simulink library "ODEsim"  (R2024b)
settings: Solver=VariableStepAuto  StartTime=0.0  StopTime=10.0  RelTol=1e-3
undefined symbols (not defined in the file or in its folder): Cline_2, Cline_r_2, Cout_9, Fb_18, Fb_d_18, fs_9, K_d_18, Ki_18, Ki_4, Kp_18, Kp_4, Len_2, R_4, r_C, r_C_1, Rline_2, Rload, Td_18, Td_4
libraries: fl_lib x97, ee_lib x24, nesl_utility x20, simulink_extras x2, spsSawtoothGeneratorLib x2, simulink x2
(part 2 of 2)

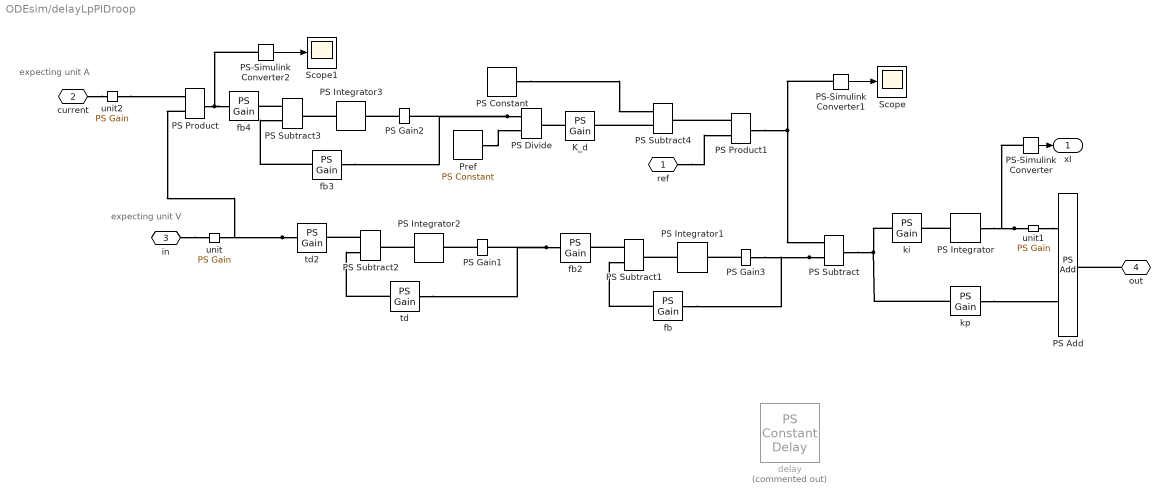
== system ODEsim/delayLpPIDroop ==
  note: expecting unit A
  note: expecting unit V
  K_d : fl_lib/Physical Signals/Functions/PS Gain  gain=K_d_18
  PS Add : fl_lib/Physical Signals/Functions/PS Add
  PS Constant : fl_lib/Physical Signals/Sources/PS Constant  constant=1
  PS Divide : fl_lib/Physical Signals/Functions/PS Divide
  PS Gain1 : fl_lib/Physical Signals/Functions/PS Gain  gain=1 1/s
  PS Gain2 : fl_lib/Physical Signals/Functions/PS Gain  gain=1 1/s
  PS Gain3 : fl_lib/Physical Signals/Functions/PS Gain  gain=1 1/s
  PS Integrator : fl_lib/Physical Signals/Linear Operators/PS Integrator  reset_method=foundation.enum.IntegratorResetSpec.None  initial_condition_spec=foundation.enum.IntegratorICSpec.Internal  saturation_spec=foundation.enum.IntegratorSaturationSpec.Both  saturation_source_spec=foundation.enum.IntegratorSaturationSourceSpec.Internal  x0=0 s  xu=90 s  xl=-0 s
  PS Integrator1 : fl_lib/Physical Signals/Linear Operators/PS Integrator  reset_method=foundation.enum.IntegratorResetSpec.None  initial_condition_spec=foundation.enum.IntegratorICSpec.Internal  saturation_spec=foundation.enum.IntegratorSaturationSpec.None  saturation_source_spec=foundation.enum.IntegratorSaturationSourceSpec.Internal  x0=0 s  xu=inf s  xl=-inf s
  PS Integrator2 : fl_lib/Physical Signals/Linear Operators/PS Integrator  reset_method=foundation.enum.IntegratorResetSpec.None  initial_condition_spec=foundation.enum.IntegratorICSpec.Internal  saturation_spec=foundation.enum.IntegratorSaturationSpec.None  saturation_source_spec=foundation.enum.IntegratorSaturationSourceSpec.Internal  x0=0 s  xu=inf s  xl=-inf s
  PS Integrator3 : fl_lib/Physical Signals/Linear Operators/PS Integrator  reset_method=foundation.enum.IntegratorResetSpec.None  initial_condition_spec=foundation.enum.IntegratorICSpec.Internal  saturation_spec=foundation.enum.IntegratorSaturationSpec.None  saturation_source_spec=foundation.enum.IntegratorSaturationSourceSpec.Internal  x0=0 s  xu=inf s  xl=-inf s
  PS Product : fl_lib/Physical Signals/Functions/PS Product
  PS Product1 : fl_lib/Physical Signals/Functions/PS Product
  PS Subtract{,1..4} (5 alike) : fl_lib/Physical Signals/Functions/PS Subtract
  PS-Simulink Converter : nesl_utility/PS-Simulink Converter  PhysicalDomain=network_engine_domain  SubClassName=ps_output  LeftPortType=input  RightPortType=output  PseudoPeriodic=off  Frequencies=[]  VectorFormat=inherit  Unit=inherit  AffineConversion=off
  PS-Simulink Converter1 : nesl_utility/PS-Simulink Converter  PhysicalDomain=network_engine_domain  SubClassName=ps_output  LeftPortType=input  RightPortType=output  PseudoPeriodic=off  Frequencies=[]  VectorFormat=inherit  Unit=inherit  AffineConversion=off
  PS-Simulink Converter2 : nesl_utility/PS-Simulink Converter  PhysicalDomain=network_engine_domain  SubClassName=ps_output  LeftPortType=input  RightPortType=output  PseudoPeriodic=off  Frequencies=[]  VectorFormat=inherit  Unit=inherit  AffineConversion=off
  Pref : fl_lib/Physical Signals/Sources/PS Constant  constant=P_d_18
  Scope : Scope
  Scope1 : Scope
  delay : fl_lib/Physical Signals/Delays/PS Constant Delay  Commented=on  InputHistory=0.0  DelayTime=Td_4 s
      settings: InternalSimscapePortConfiguration="{\"Bottom\":[],\"Left\":[{\"id\":\"U\",\"label\":\"U\",\"type\":\"input\"}],\"Right\":[{\"id\":\"Y\",\"label\":\"Y\",\"type\":\"output\"}],\"Top\":[]}"
  fb : fl_lib/Physical Signals/Functions/PS Gain  gain=2*pi*Fb_18
  fb2 : fl_lib/Physical Signals/Functions/PS Gain  gain=2*pi*Fb_18
  fb3 : fl_lib/Physical Signals/Functions/PS Gain  gain=Fb_d_18* 2 * pi
  fb4 : fl_lib/Physical Signals/Functions/PS Gain  gain=Fb_d_18* 2 * pi
  ki : fl_lib/Physical Signals/Functions/PS Gain  gain=Ki_18
  kp : fl_lib/Physical Signals/Functions/PS Gain  gain=Kp_18
  td : fl_lib/Physical Signals/Functions/PS Gain  gain=1/Td_18
  td2 : fl_lib/Physical Signals/Functions/PS Gain  gain=1/Td_18
  unit : fl_lib/Physical Signals/Functions/PS Gain  gain=1 1/V
  unit1 : fl_lib/Physical Signals/Functions/PS Gain  gain=1 1/s
  unit2 : fl_lib/Physical Signals/Functions/PS Gain  gain=1 1/A
  ref : PMIOPort  Side=Left
  current : PMIOPort  Port=2  Side=Left
  in : PMIOPort  Port=3  Side=Left
  out : PMIOPort  Port=4  Side=Right
  xI : Outport
  wires:
  PS-Simulink Converter/1 -> xI/1
  PS-Simulink Converter1/1 -> Scope/1
  PS-Simulink Converter2/1 -> Scope1/1
  connections:
  PS Subtract4/LConn2 -- K_d/RConn1
  PS Product1/RConn1 -- PS Subtract/LConn1 -- PS-Simulink Converter1/LConn1
  ref/RConn1 -- PS Product1/LConn2
  PS Product1/LConn1 -- PS Subtract4/RConn1
  Pref/RConn1 -- PS Divide/LConn2
  PS Constant/RConn1 -- PS Subtract4/LConn1
  K_d/LConn1 -- PS Divide/RConn1
  unit2/RConn1 -- PS Product/LConn1
  current/RConn1 -- unit2/LConn1
  fb3/RConn1 -- PS Subtract3/LConn2
  PS Subtract3/LConn1 -- fb4/RConn1
  PS Integrator3/LConn1 -- PS Subtract3/RConn1
  PS Gain2/LConn1 -- PS Integrator3/RConn1
  PS Product/RConn1 -- PS-Simulink Converter2/LConn1 -- fb4/LConn1
  PS Divide/LConn1 -- PS Gain2/RConn1 -- fb3/LConn1
  td/RConn1 -- PS Subtract2/LConn2
  PS Integrator2/LConn1 -- PS Subtract2/RConn1
  PS Subtract2/LConn1 -- td2/RConn1
  PS Gain1/LConn1 -- PS Integrator2/RConn1
  td2/LConn1 -- unit/RConn1 -- PS Product/LConn2
  fb2/LConn1 -- PS Gain1/RConn1 -- td/LConn1
  unit1/RConn1 -- PS Add/LConn1
  PS Subtract/RConn1 -- kp/LConn1 -- ki/LConn1
  PS Integrator/LConn1 -- ki/RConn1
  in/RConn1 -- unit/LConn1
  unit1/LConn1 -- PS Integrator/RConn1 -- PS-Simulink Converter/LConn1
  kp/RConn1 -- PS Add/LConn2
  out/RConn1 -- PS Add/RConn1
  PS Subtract/LConn2 -- PS Gain3/RConn1 -- fb/LConn1
  fb/RConn1 -- PS Subtract1/LConn2
  PS Integrator1/LConn1 -- PS Subtract1/RConn1
  PS Subtract1/LConn1 -- fb2/RConn1
  PS Gain3/LConn1 -- PS Integrator1/RConn1

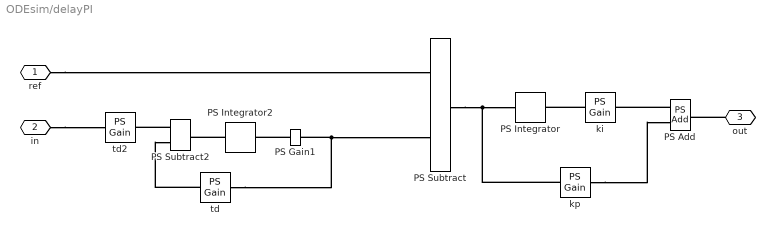
== system ODEsim/delayPI ==
  PS Add : fl_lib/Physical Signals/Functions/PS Add
  PS Gain1 : fl_lib/Physical Signals/Functions/PS Gain  gain=1 1/s
  PS Integrator : fl_lib/Physical Signals/Linear Operators/PS Integrator  reset_method=foundation.enum.IntegratorResetSpec.None  initial_condition_spec=foundation.enum.IntegratorICSpec.Internal  saturation_spec=foundation.enum.IntegratorSaturationSpec.None  saturation_source_spec=foundation.enum.IntegratorSaturationSourceSpec.Internal  x0=0 s  xu=inf s  xl=-inf s
  PS Integrator2 : fl_lib/Physical Signals/Linear Operators/PS Integrator  reset_method=foundation.enum.IntegratorResetSpec.None  initial_condition_spec=foundation.enum.IntegratorICSpec.Internal  saturation_spec=foundation.enum.IntegratorSaturationSpec.None  saturation_source_spec=foundation.enum.IntegratorSaturationSourceSpec.Internal  x0=0 s  xu=inf s  xl=-inf s
  PS Subtract : fl_lib/Physical Signals/Functions/PS Subtract
  PS Subtract2 : fl_lib/Physical Signals/Functions/PS Subtract
  ki : fl_lib/Physical Signals/Functions/PS Gain  gain=Ki_4 1/s
  kp : fl_lib/Physical Signals/Functions/PS Gain  gain=Kp_4
  td : fl_lib/Physical Signals/Functions/PS Gain  gain=1/Td_18
  td2 : fl_lib/Physical Signals/Functions/PS Gain  gain=1/Td_18
  ref : PMIOPort  Side=Left
  in : PMIOPort  Port=2  Side=Left
  out : PMIOPort  Port=3  Side=Right
  connections:
  out/RConn1 -- PS Add/RConn1
  kp/RConn1 -- PS Add/LConn2
  ki/LConn1 -- PS Integrator/RConn1
  PS Add/LConn1 -- ki/RConn1
  in/RConn1 -- td2/LConn1
  td/LConn1 -- PS Subtract/LConn2 -- PS Gain1/RConn1
  ref/RConn1 -- PS Subtract/LConn1
  PS Subtract/RConn1 -- kp/LConn1 -- PS Integrator/LConn1
  td/RConn1 -- PS Subtract2/LConn2
  PS Subtract2/LConn1 -- td2/RConn1
  PS Integrator2/LConn1 -- PS Subtract2/RConn1
  PS Gain1/LConn1 -- PS Integrator2/RConn1

== system ODEsim/loadRL ==
  Lload : ee_lib/Passive/Inductor  l=Lload H  enable_L_tol=ee.enum.toleranceApplication.none  L_tol=20  tol_distribution=ee.enum.toleranceDistribution.uniform  nSigma=4  r=0 Ohm  g=0 1/Ohm  enable_operating_limits=ee.enum.enable.no  operating_limit_action=ee.enum.passive.reportOpLim.warn  max_working_current=1 A  power_rating=1 W  fault_action=simscape.enum.assert.action.none  t_fault=1 s  i_L_specify=off  i_L_priority=High  i_L=0 A  i_L_nominal_specify=off  i_L_nominal_value=1  i_L_nominal_unit=A
  M : Subsystem
      settings: CopyFcn=set_param(gcb,'LinkStatus','none')  PortSchema="{\"entries\":[{\"content\":{\"sides\":[{\"content\":{\"connectorIds\":[\"LConn1\"]},\"type\":\"ConnectorPlacement.EquallySpacedRectSide\",\"uuid\":\"40852030-531f-4f43-a55b-e3170444f81a\"},{\"content\":{\"connectorIds\":[\"RConn1\"],\"side\":\"RIGHT\"},\"type\":\"ConnectorPlacement.EquallySpacedRectSide\",\"uuid\":\"1f30083b-b568-47ae-a4c9-b443d22c2592\"},{\"content\":{\"connectorIds\":[\"LConn2\"],\"side\":\"TOP\"},\"type\":\"ConnectorPlacement.EquallySpacedRectSide\",\"uuid\":\"3c071041-7a52-4d22-9e74-6a603f214a57\"}]},\"type\":\"ConnectorPlacement.EquallySpacedConnector\",\"uuid\":\"06d852a0-3ad3-4e59-bc5b-9ea8903862cb\"}],\"packageUris\":[\"http://schema.mathworks.com/mf0/Connector/R2020b\"],\"version\":\"1.0\"}"
  Rload : fl_lib/Electrical/Electrical Elements/Resistor  R=Rload Ohm  i_specify=off  i_priority=None  i=0 A  i_nominal_specify=off  i_nominal_value=1  i_nominal_unit=A  v_specify=off  v_priority=None  v=0 V  v_nominal_specify=off  v_nominal_value=1  v_nominal_unit=V
  In : PMIOPort  Side=Left
  Gnd : PMIOPort  Port=2  Side=Left
  i_L : PMIOPort  Port=3  Side=Left
  connections:
  Gnd/RConn1 -- M/RConn1
  Rload/LConn1 -- In/RConn1
  M/LConn1 -- Lload/RConn1
  Rload/RConn1 -- Lload/LConn1
  i_L/RConn1 -- M/LConn2

== system ODEsim/loadVarRL ==
  Lload : ee_lib/Passive/Inductor  l=Lload_3 H  enable_L_tol=ee.enum.toleranceApplication.none  L_tol=20  tol_distribution=ee.enum.toleranceDistribution.uniform  nSigma=4  r=0 Ohm  g=0 1/Ohm  enable_operating_limits=ee.enum.enable.no  operating_limit_action=ee.enum.passive.reportOpLim.warn  max_working_current=1 A  power_rating=1 W  fault_action=simscape.enum.assert.action.none  t_fault=1 s  i_L_specify=off  i_L_priority=High  i_L=0 A  i_L_nominal_specify=off  i_L_nominal_value=1  i_L_nominal_unit=A
  M : Subsystem
      settings: CopyFcn=set_param(gcb,'LinkStatus','none')  PortSchema="{\"entries\":[{\"content\":{\"sides\":[{\"content\":{\"connectorIds\":[\"LConn1\"]},\"type\":\"ConnectorPlacement.EquallySpacedRectSide\",\"uuid\":\"40852030-531f-4f43-a55b-e3170444f81a\"},{\"content\":{\"connectorIds\":[\"RConn1\"],\"side\":\"RIGHT\"},\"type\":\"ConnectorPlacement.EquallySpacedRectSide\",\"uuid\":\"1f30083b-b568-47ae-a4c9-b443d22c2592\"},{\"content\":{\"connectorIds\":[\"LConn2\"],\"side\":\"TOP\"},\"type\":\"ConnectorPlacement.EquallySpacedRectSide\",\"uuid\":\"3c071041-7a52-4d22-9e74-6a603f214a57\"}]},\"type\":\"ConnectorPlacement.EquallySpacedConnector\",\"uuid\":\"06d852a0-3ad3-4e59-bc5b-9ea8903862cb\"}],\"packageUris\":[\"http://schema.mathworks.com/mf0/Connector/R2020b\"],\"version\":\"1.0\"}"
  Variable Resistor : fl_lib/Electrical/Electrical Elements/Variable Resistor  Rmin=0 Ohm  thermalEnable=false  thermal_mass=1 J/K  i_specify=off  i_priority=None  i=0 A  i_nominal_specify=off  i_nominal_value=1  i_nominal_unit=A  v_specify=off  v_priority=None  v=0 V  v_nominal_specify=off  v_nominal_value=1  v_nominal_unit=V  T_specify=off  T_priority=None  T=300 K  T_nominal_specify=off  T_nominal_value=1  T_nominal_unit=K
  In : PMIOPort  Side=Left
  Gnd : PMIOPort  Port=2  Side=Left
  i_L : PMIOPort  Port=3  Side=Left
  R : PMIOPort  Port=4  Side=Right
  connections:
  Lload/LConn1 -- Variable Resistor/RConn1
  Lload/RConn1 -- M/LConn1
  R/RConn1 -- Variable Resistor/LConn1
  In/RConn1 -- Variable Resistor/LConn2
  M/RConn1 -- Gnd/RConn1
  i_L/RConn1 -- M/LConn2

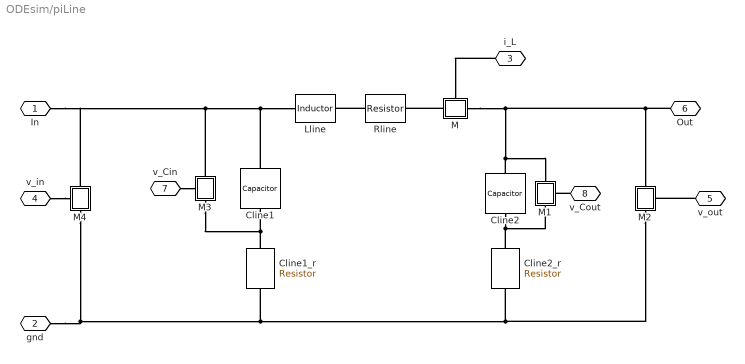
== system ODEsim/piLine ==
  Cline1 : fl_lib/Electrical/Electrical Elements/Capacitor  c=Cline_2 / 2 *Len_2 F  r=0 Ohm  g=0 1/Ohm  i_specify=off  i_priority=None  i=0 A  i_nominal_specify=off  i_nominal_value=1  i_nominal_unit=A  v_specify=off  v_priority=None  v=0 V  v_nominal_specify=off  v_nominal_value=1  v_nominal_unit=V  vc_specify=off  vc_priority=High  vc=0 V  vc_nominal_specify=off  vc_nominal_value=1  vc_nominal_unit=V
  Cline1_r : fl_lib/Electrical/Electrical Elements/Resistor  R=Cline_r_2 Ohm  i_specify=off  i_priority=None  i=0 A  i_nominal_specify=off  i_nominal_value=1  i_nominal_unit=A  v_specify=off  v_priority=None  v=0 V  v_nominal_specify=off  v_nominal_value=1  v_nominal_unit=V
  Cline2 : fl_lib/Electrical/Electrical Elements/Capacitor  c=Cline_2 / 2 *Len_2 F  r=0 Ohm  g=0 1/Ohm  i_specify=off  i_priority=None  i=0 A  i_nominal_specify=off  i_nominal_value=1  i_nominal_unit=A  v_specify=off  v_priority=None  v=0 V  v_nominal_specify=off  v_nominal_value=1  v_nominal_unit=V  vc_specify=off  vc_priority=High  vc=0 V  vc_nominal_specify=off  vc_nominal_value=1  vc_nominal_unit=V
  Cline2_r : fl_lib/Electrical/Electrical Elements/Resistor  R=Cline_r_2 Ohm  i_specify=off  i_priority=None  i=0 A  i_nominal_specify=off  i_nominal_value=1  i_nominal_unit=A  v_specify=off  v_priority=None  v=0 V  v_nominal_specify=off  v_nominal_value=1  v_nominal_unit=V
  Lline : fl_lib/Electrical/Electrical Elements/Inductor  l=Lline_2 H  r=0 Ohm  g=0 1/Ohm  i_specify=off  i_priority=None  i=0 A  i_nominal_specify=off  i_nominal_value=1  i_nominal_unit=A  v_specify=off  v_priority=None  v=0 V  v_nominal_specify=off  v_nominal_value=1  v_nominal_unit=V  i_L_specify=off  i_L_priority=High  i_L=0 A  i_L_nominal_specify=off  i_L_nominal_value=1  i_L_nominal_unit=A
  M : Subsystem
      settings: CopyFcn=set_param(gcb,'LinkStatus','none')  PortSchema="{\"entries\":[{\"content\":{\"sides\":[{\"content\":{\"connectorIds\":[\"LConn1\"]},\"type\":\"ConnectorPlacement.EquallySpacedRectSide\",\"uuid\":\"40852030-531f-4f43-a55b-e3170444f81a\"},{\"content\":{\"connectorIds\":[\"RConn1\"],\"side\":\"RIGHT\"},\"type\":\"ConnectorPlacement.EquallySpacedRectSide\",\"uuid\":\"1f30083b-b568-47ae-a4c9-b443d22c2592\"},{\"content\":{\"connectorIds\":[\"LConn2\"],\"side\":\"TOP\"},\"type\":\"ConnectorPlacement.EquallySpacedRectSide\",\"uuid\":\"3c071041-7a52-4d22-9e74-6a603f214a57\"}]},\"type\":\"ConnectorPlacement.EquallySpacedConnector\",\"uuid\":\"06d852a0-3ad3-4e59-bc5b-9ea8903862cb\"}],\"packageUris\":[\"http://schema.mathworks.com/mf0/Connector/R2020b\"],\"version\":\"1.0\"}"
  M1 : Subsystem
      settings: CopyFcn=set_param(gcb,'LinkStatus','none')  PortSchema="{\"entries\":[{\"content\":{\"sides\":[{\"content\":{\"connectorIds\":[\"LConn1\"]},\"type\":\"ConnectorPlacement.EquallySpacedRectSide\",\"uuid\":\"06c3c841-7f27-414f-b368-a176494b6f9d\"},{\"content\":{\"connectorIds\":[\"RConn1\"],\"side\":\"RIGHT\"},\"type\":\"ConnectorPlacement.EquallySpacedRectSide\",\"uuid\":\"1b123208-a0a4-432d-8d9c-871fed45b507\"},{\"content\":{\"connectorIds\":[\"LConn2\"],\"side\":\"TOP\"},\"type\":\"ConnectorPlacement.EquallySpacedRectSide\",\"uuid\":\"cfe0dd68-fe1a-447a-9562-3abbfb037eea\"}]},\"type\":\"ConnectorPlacement.EquallySpacedConnector\",\"uuid\":\"2a5dcc2a-148a-4bfc-a97a-46b06b110d1b\"}],\"packageUris\":[\"http://schema.mathworks.com/mf0/Connector/R2020b\"],\"version\":\"1.0\"}"
  M2 : Subsystem
      settings: CopyFcn=set_param(gcb,'LinkStatus','none')  PortSchema="{\"entries\":[{\"content\":{\"sides\":[{\"content\":{\"connectorIds\":[\"LConn1\"]},\"type\":\"ConnectorPlacement.EquallySpacedRectSide\",\"uuid\":\"06c3c841-7f27-414f-b368-a176494b6f9d\"},{\"content\":{\"connectorIds\":[\"RConn1\"],\"side\":\"RIGHT\"},\"type\":\"ConnectorPlacement.EquallySpacedRectSide\",\"uuid\":\"1b123208-a0a4-432d-8d9c-871fed45b507\"},{\"content\":{\"connectorIds\":[\"LConn2\"],\"side\":\"TOP\"},\"type\":\"ConnectorPlacement.EquallySpacedRectSide\",\"uuid\":\"cfe0dd68-fe1a-447a-9562-3abbfb037eea\"}]},\"type\":\"ConnectorPlacement.EquallySpacedConnector\",\"uuid\":\"2a5dcc2a-148a-4bfc-a97a-46b06b110d1b\"}],\"packageUris\":[\"http://schema.mathworks.com/mf0/Connector/R2020b\"],\"version\":\"1.0\"}"
  M3 : Subsystem
      settings: CopyFcn=set_param(gcb,'LinkStatus','none')  PortSchema="{\"entries\":[{\"content\":{\"sides\":[{\"content\":{\"connectorIds\":[\"LConn1\"]},\"type\":\"ConnectorPlacement.EquallySpacedRectSide\",\"uuid\":\"06c3c841-7f27-414f-b368-a176494b6f9d\"},{\"content\":{\"connectorIds\":[\"RConn1\"],\"side\":\"RIGHT\"},\"type\":\"ConnectorPlacement.EquallySpacedRectSide\",\"uuid\":\"1b123208-a0a4-432d-8d9c-871fed45b507\"},{\"content\":{\"connectorIds\":[\"LConn2\"],\"side\":\"TOP\"},\"type\":\"ConnectorPlacement.EquallySpacedRectSide\",\"uuid\":\"cfe0dd68-fe1a-447a-9562-3abbfb037eea\"}]},\"type\":\"ConnectorPlacement.EquallySpacedConnector\",\"uuid\":\"2a5dcc2a-148a-4bfc-a97a-46b06b110d1b\"}],\"packageUris\":[\"http://schema.mathworks.com/mf0/Connector/R2020b\"],\"version\":\"1.0\"}"
  M4 : Subsystem
      settings: CopyFcn=set_param(gcb,'LinkStatus','none')  PortSchema="{\"entries\":[{\"content\":{\"sides\":[{\"content\":{\"connectorIds\":[\"LConn1\"]},\"type\":\"ConnectorPlacement.EquallySpacedRectSide\",\"uuid\":\"06c3c841-7f27-414f-b368-a176494b6f9d\"},{\"content\":{\"connectorIds\":[\"RConn1\"],\"side\":\"RIGHT\"},\"type\":\"ConnectorPlacement.EquallySpacedRectSide\",\"uuid\":\"1b123208-a0a4-432d-8d9c-871fed45b507\"},{\"content\":{\"connectorIds\":[\"LConn2\"],\"side\":\"TOP\"},\"type\":\"ConnectorPlacement.EquallySpacedRectSide\",\"uuid\":\"cfe0dd68-fe1a-447a-9562-3abbfb037eea\"}]},\"type\":\"ConnectorPlacement.EquallySpacedConnector\",\"uuid\":\"2a5dcc2a-148a-4bfc-a97a-46b06b110d1b\"}],\"packageUris\":[\"http://schema.mathworks.com/mf0/Connector/R2020b\"],\"version\":\"1.0\"}"
  Rline : fl_lib/Electrical/Electrical Elements/Resistor  R=Rline_2 Ohm  i_specify=off  i_priority=None  i=0 A  i_nominal_specify=off  i_nominal_value=1  i_nominal_unit=A  v_specify=off  v_priority=None  v=0 V  v_nominal_specify=off  v_nominal_value=1  v_nominal_unit=V
  In : PMIOPort  Side=Left
  gnd : PMIOPort  Port=2  Side=Left
  i_L : PMIOPort  Port=3  Side=Left
  v_in : PMIOPort  Port=4  Side=Left
  v_out : PMIOPort  Port=5  Side=Left
  Out : PMIOPort  Port=6  Side=Right
  v_Cin : PMIOPort  Port=7  Side=Right
  v_Cout : PMIOPort  Port=8  Side=Right
  connections:
  Cline1/LConn1 -- In/RConn1 -- M4/LConn1 -- M3/LConn1 -- Lline/LConn1
  gnd/RConn1 -- M4/RConn1 -- Cline1_r/RConn1 -- M2/RConn1 -- Cline2_r/RConn1
  Cline1_r/LConn1 -- M3/RConn1 -- Cline1/RConn1
  Cline2_r/LConn1 -- M1/RConn1 -- Cline2/RConn1
  M/LConn1 -- Rline/RConn1
  Rline/LConn1 -- Lline/RConn1
  i_L/RConn1 -- M/LConn2
  v_Cout/RConn1 -- M1/LConn2
  v_out/RConn1 -- M2/LConn2
  Out/RConn1 -- M/RConn1 -- M1/LConn1 -- Cline2/LConn1 -- M2/LConn1
  v_Cin/RConn1 -- M3/LConn2
  v_in/RConn1 -- M4/LConn2

== system ODEsim/Boost_Switching/M ==
  Current Sensor : fl_lib/Electrical/Electrical Sensors/Current Sensor
  + : PMIOPort  Side=Left
  I : PMIOPort  Port=2  Side=Left
  - : PMIOPort  Port=3  Side=Right
  connections:
  -/RConn1 -- Current Sensor/RConn2
  I/RConn1 -- Current Sensor/RConn1
  Current Sensor/LConn1 -- +/RConn1

== system ODEsim/Boost_Switching/M1 ==
  Voltage Sensor : fl_lib/Electrical/Electrical Sensors/Voltage Sensor
  + : PMIOPort  Side=Left
  v : PMIOPort  Port=2  Side=Left
  - : PMIOPort  Port=3  Side=Right
  connections:
  -/RConn1 -- Voltage Sensor/RConn2
  +/RConn1 -- Voltage Sensor/LConn1
  v/RConn1 -- Voltage Sensor/RConn1

== system ODEsim/Boost_Switching/M2 ==
  Voltage Sensor : fl_lib/Electrical/Electrical Sensors/Voltage Sensor
  + : PMIOPort  Side=Left
  v : PMIOPort  Port=2  Side=Left
  - : PMIOPort  Port=3  Side=Right
  connections:
  -/RConn1 -- Voltage Sensor/RConn2
  +/RConn1 -- Voltage Sensor/LConn1
  v/RConn1 -- Voltage Sensor/RConn1

== system ODEsim/Buck_Switching/M ==
  Current Sensor : fl_lib/Electrical/Electrical Sensors/Current Sensor
  + : PMIOPort  Side=Left
  i : PMIOPort  Port=2  Side=Left
  - : PMIOPort  Port=3  Side=Right
  connections:
  Current Sensor/LConn1 -- +/RConn1
  i/RConn1 -- Current Sensor/RConn1
  -/RConn1 -- Current Sensor/RConn2

== system ODEsim/Buck_Switching/M1 ==
  Voltage Sensor : fl_lib/Electrical/Electrical Sensors/Voltage Sensor
  + : PMIOPort  Side=Left
  v : PMIOPort  Port=2  Side=Left
  - : PMIOPort  Port=3  Side=Right
  connections:
  v/RConn1 -- Voltage Sensor/RConn1
  +/RConn1 -- Voltage Sensor/LConn1
  -/RConn1 -- Voltage Sensor/RConn2

== system ODEsim/Buck_Switching/M2 ==
  Voltage Sensor : fl_lib/Electrical/Electrical Sensors/Voltage Sensor
  + : PMIOPort  Side=Left
  v : PMIOPort  Port=2  Side=Left
  - : PMIOPort  Port=3  Side=Right
  connections:
  -/RConn1 -- Voltage Sensor/RConn2
  +/RConn1 -- Voltage Sensor/LConn1
  v/RConn1 -- Voltage Sensor/RConn1

== system ODEsim/DAB_Switching/M1 ==
  Voltage Sensor : fl_lib/Electrical/Electrical Sensors/Voltage Sensor
  + : PMIOPort  Side=Left
  v : PMIOPort  Port=2  Side=Left
  - : PMIOPort  Port=3  Side=Right
  connections:
  +/RConn1 -- Voltage Sensor/LConn1
  -/RConn1 -- Voltage Sensor/RConn2
  v/RConn1 -- Voltage Sensor/RConn1

== system ODEsim/DAB_Switching/M2 ==
  Current Sensor : fl_lib/Electrical/Electrical Sensors/Current Sensor
  + : PMIOPort  Side=Left
  i : PMIOPort  Port=2  Side=Left
  - : PMIOPort  Port=3  Side=Right
  connections:
  -/RConn1 -- Current Sensor/RConn2
  i/RConn1 -- Current Sensor/RConn1
  Current Sensor/LConn1 -- +/RConn1

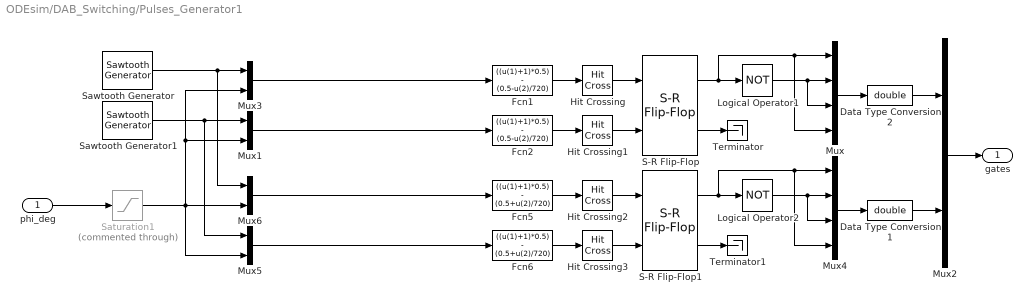
== system ODEsim/DAB_Switching/Pulses_Generator1 ==
  phi_deg : Inport
  Data Type Conversion1 : DataTypeConversion  OutDataTypeStr=double  SaturateOnIntegerOverflow=off  RndMeth=Floor
  Data Type Conversion2 : DataTypeConversion  OutDataTypeStr=double  SaturateOnIntegerOverflow=off  RndMeth=Floor
  Fcn1 : Fcn  Expr=((u(1)+1)*0.5) - (0.5-u(2)/720)
  Fcn2 : Fcn  Expr=((u(1)+1)*0.5) - (0.5-u(2)/720)
  Fcn5 : Fcn  Expr=((u(1)+1)*0.5) - (0.5+u(2)/720)
  Fcn6 : Fcn  Expr=((u(1)+1)*0.5) - (0.5+u(2)/720)
  Hit Crossing{,1..3} (4 alike) : HitCross  HitCrossingDirection=rising
  Logical Operator1 : Logic  Operator=NOT  AllPortsSameDT=off  OutDataTypeStr=boolean
  Logical Operator2 : Logic  Operator=NOT  AllPortsSameDT=off  OutDataTypeStr=boolean
  Mux : Mux
  Mux{1,3,5..6} (4 alike) : Mux  Inputs=2
  Mux2 : Mux  Inputs=[4,4]
  Mux4 : Mux
  S-R Flip-Flop : simulink_extras/Flip Flops/S-R Flip-Flop  initial_condition=0
  S-R Flip-Flop1 : simulink_extras/Flip Flops/S-R Flip-Flop  initial_condition=0
  Saturation1 : Saturate  Commented=through  UpperLimit=180  LowerLimit=-180
  Sawtooth Generator : spsSawtoothGeneratorLib/Sawtooth Generator  Freq=fs  Phase=0  Ts=0
  Sawtooth Generator1 : spsSawtoothGeneratorLib/Sawtooth Generator  Freq=fs  Phase=180  Ts=0
  Terminator : Terminator
  Terminator1 : Terminator
  gates : Outport
  wires:
  Logical Operator2/1 -> Mux4/2, Mux4/3
  Fcn5/1 -> Hit Crossing2/1
  Fcn6/1 -> Hit Crossing3/1
  Hit Crossing2/1 -> S-R Flip-Flop1/1
  Hit Crossing3/1 -> S-R Flip-Flop1/2
  S-R Flip-Flop1/1 -> Mux4/4, Mux4/1, Logical Operator2/1
  S-R Flip-Flop1/2 -> Terminator1/1
  Mux4/1 -> Data Type Conversion1/1
  Mux6/1 -> Fcn5/1
  Mux5/1 -> Fcn6/1
  Saturation1/1 -> Mux3/2, Mux1/2, Mux5/2, Mux6/2
  Sawtooth Generator1/1 -> Mux1/1, Mux5/1
  Mux1/1 -> Fcn2/1
  Mux3/1 -> Fcn1/1
  Data Type Conversion1/1 -> Mux2/2
  Data Type Conversion2/1 -> Mux2/1
  Mux/1 -> Data Type Conversion2/1
  S-R Flip-Flop/2 -> Terminator/1
  S-R Flip-Flop/1 -> Logical Operator1/1, Mux/1, Mux/4
  Hit Crossing1/1 -> S-R Flip-Flop/2
  Hit Crossing/1 -> S-R Flip-Flop/1
  Fcn2/1 -> Hit Crossing1/1
  Fcn1/1 -> Hit Crossing/1
  Sawtooth Generator/1 -> Mux3/1, Mux6/1
  phi_deg/1 -> Saturation1/1
  Logical Operator1/1 -> Mux/3, Mux/2
  Mux2/1 -> gates/1

== system ODEsim/dabGAM/Cout ==
  note: Current Sensor3
  note: It is easy to get algebraic loops when using simulink and simscape. For inductors and capacitors, it can be easy to bypass this by integrating for the other state in Simulink instead of taking it directly from Simscape. This could introduce error of very long simulations
  C_out : fl_lib/Electrical/Electrical Elements/Capacitor  c=C F  r=0 Ohm  g=0 1/Ohm  i_specify=off  i_priority=None  i=0 A  i_nominal_specify=off  i_nominal_value=1  i_nominal_unit=A  v_specify=off  v_priority=None  v=0 V  v_nominal_specify=off  v_nominal_value=1  v_nominal_unit=V  vc_specify=on  vc_priority=High  vc=V0 V  vc_nominal_specify=off  vc_nominal_value=1  vc_nominal_unit=V
  Current Sensor : fl_lib/Electrical/Electrical Sensors/Current Sensor
  PS Gain : fl_lib/Physical Signals/Functions/PS Gain  gain=1/C 1/A
  PS Gain1 : fl_lib/Physical Signals/Functions/PS Gain  gain=1 V/s
  PS Integrator : fl_lib/Physical Signals/Linear Operators/PS Integrator  reset_method=foundation.enum.IntegratorResetSpec.None  initial_condition_spec=foundation.enum.IntegratorICSpec.Internal  saturation_spec=foundation.enum.IntegratorSaturationSpec.None  saturation_source_spec=foundation.enum.IntegratorSaturationSourceSpec.Internal  x0=V0 s  xu=inf s  xl=-inf s
  + : PMIOPort  Side=Left
  - : PMIOPort  Port=2  Side=Right
  Voltage : PMIOPort  Port=3  Side=Right
  connections:
  PS Gain/LConn1 -- Current Sensor/RConn1
  C_out/RConn1 -- -/RConn1
  Current Sensor/LConn1 -- +/RConn1
  Current Sensor/RConn2 -- C_out/LConn1
  PS Integrator/LConn1 -- PS Gain/RConn1
  PS Gain1/RConn1 -- Voltage/RConn1
  PS Integrator/RConn1 -- PS Gain1/LConn1

== system ODEsim/dabGAM/M2 ==
  Current Sensor : fl_lib/Electrical/Electrical Sensors/Current Sensor
  + : PMIOPort  Side=Left
  i : PMIOPort  Port=2  Side=Left
  - : PMIOPort  Port=3  Side=Right
  connections:
  -/RConn1 -- Current Sensor/RConn2
  i/RConn1 -- Current Sensor/RConn1
  Current Sensor/LConn1 -- +/RConn1

== system ODEsim/dabGAM/M3 ==
  Voltage Sensor : fl_lib/Electrical/Electrical Sensors/Voltage Sensor
  + : PMIOPort  Side=Left
  - : PMIOPort  Port=2  Side=Right
  v : PMIOPort  Port=3  Side=Right
  connections:
  v/RConn1 -- Voltage Sensor/RConn1
  -/RConn1 -- Voltage Sensor/RConn2
  +/RConn1 -- Voltage Sensor/LConn1

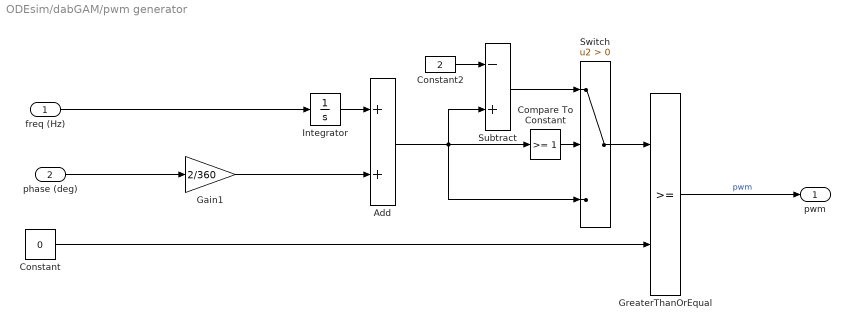
== system ODEsim/dabGAM/pwm generator ==
  freq (Hz) : Inport
  phase (deg) : Inport  Port=2
  Add : Sum
  Compare To Constant : simulink/Logic and Bit Operations/Compare To Constant  relop=>=  const=1  OutDataTypeStr=boolean
  Constant : Constant  Value=0
  Constant2 : Constant  Value=2
  Gain1 : Gain  Gain=2/360
  GreaterThanOrEqual : RelationalOperator  OutDataTypeStr=boolean  RndMeth=Simplest  InputSameDT=off
  Integrator : Integrator  WrapState=on  WrappedStateUpperValue=1  WrappedStateLowerValue=-1
  Subtract : Sum  Inputs=-+
  Switch : Switch  Criteria=u2 > Threshold  SaturateOnIntegerOverflow=off  InputSameDT=off
  pwm : Outport
  wires:
  Constant2/1 -> Subtract/1
  Gain1/1 -> Add/2
  freq (Hz)/1 -> Integrator/1
  Constant/1 -> GreaterThanOrEqual/2
  Add/1 -> Switch/3, Subtract/2, Compare To Constant/1
  Integrator/1 -> Add/1
  Compare To Constant/1 -> Switch/2
  Subtract/1 -> Switch/1
  Switch/1 -> GreaterThanOrEqual/1
  phase (deg)/1 -> Gain1/1
  GreaterThanOrEqual/1 -> pwm/1  "pwm"

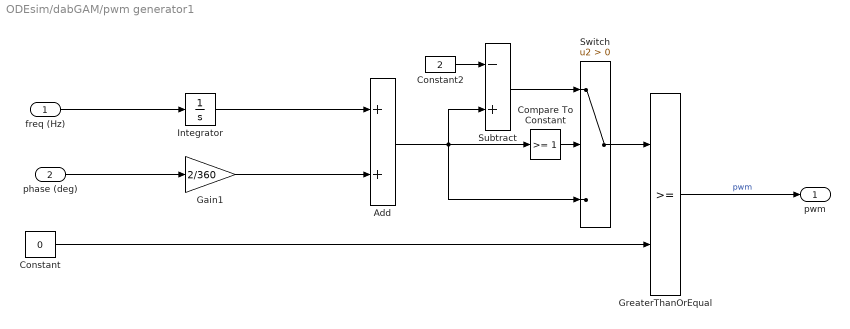
== system ODEsim/dabGAM/pwm generator1 ==
  freq (Hz) : Inport
  phase (deg) : Inport  Port=2
  Add : Sum
  Compare To Constant : simulink/Logic and Bit Operations/Compare To Constant  relop=>=  const=1  OutDataTypeStr=boolean
  Constant : Constant  Value=0
  Constant2 : Constant  Value=2
  Gain1 : Gain  Gain=2/360
  GreaterThanOrEqual : RelationalOperator  OutDataTypeStr=boolean  RndMeth=Simplest  InputSameDT=off
  Integrator : Integrator  WrapState=on  WrappedStateUpperValue=1  WrappedStateLowerValue=-1
  Subtract : Sum  Inputs=-+
  Switch : Switch  Criteria=u2 > Threshold  SaturateOnIntegerOverflow=off  InputSameDT=off
  pwm : Outport
  wires:
  GreaterThanOrEqual/1 -> pwm/1  "pwm"
  phase (deg)/1 -> Gain1/1
  Switch/1 -> GreaterThanOrEqual/1
  Subtract/1 -> Switch/1
  Compare To Constant/1 -> Switch/2
  Integrator/1 -> Add/1
  Add/1 -> Compare To Constant/1, Subtract/2, Switch/3
  Constant/1 -> GreaterThanOrEqual/2
  freq (Hz)/1 -> Integrator/1
  Gain1/1 -> Add/2
  Constant2/1 -> Subtract/1

== system ODEsim/loadRL/M ==
  Current Sensor : fl_lib/Electrical/Electrical Sensors/Current Sensor
  + : PMIOPort  Side=Left
  i : PMIOPort  Port=2  Side=Left
  - : PMIOPort  Port=3  Side=Right
  connections:
  Current Sensor/LConn1 -- +/RConn1
  i/RConn1 -- Current Sensor/RConn1
  -/RConn1 -- Current Sensor/RConn2

== system ODEsim/loadVarRL/M ==
  Current Sensor : fl_lib/Electrical/Electrical Sensors/Current Sensor
  + : PMIOPort  Side=Left
  i : PMIOPort  Port=2  Side=Left
  - : PMIOPort  Port=3  Side=Right
  connections:
  Current Sensor/LConn1 -- +/RConn1
  i/RConn1 -- Current Sensor/RConn1
  -/RConn1 -- Current Sensor/RConn2

== system ODEsim/piLine/M ==
  Current Sensor : fl_lib/Electrical/Electrical Sensors/Current Sensor
  + : PMIOPort  Side=Left
  i : PMIOPort  Port=2  Side=Left
  - : PMIOPort  Port=3  Side=Right
  connections:
  Current Sensor/LConn1 -- +/RConn1
  i/RConn1 -- Current Sensor/RConn1
  -/RConn1 -- Current Sensor/RConn2

== system ODEsim/piLine/M1 ==
  Voltage Sensor : fl_lib/Electrical/Electrical Sensors/Voltage Sensor
  + : PMIOPort  Side=Left
  v : PMIOPort  Port=2  Side=Left
  - : PMIOPort  Port=3  Side=Right
  connections:
  v/RConn1 -- Voltage Sensor/RConn1
  +/RConn1 -- Voltage Sensor/LConn1
  -/RConn1 -- Voltage Sensor/RConn2

== system ODEsim/piLine/M2 ==
  Voltage Sensor : fl_lib/Electrical/Electrical Sensors/Voltage Sensor
  + : PMIOPort  Side=Left
  v : PMIOPort  Port=2  Side=Left
  - : PMIOPort  Port=3  Side=Right
  connections:
  -/RConn1 -- Voltage Sensor/RConn2
  +/RConn1 -- Voltage Sensor/LConn1
  v/RConn1 -- Voltage Sensor/RConn1

== system ODEsim/piLine/M3 ==
  Voltage Sensor : fl_lib/Electrical/Electrical Sensors/Voltage Sensor
  + : PMIOPort  Side=Left
  v : PMIOPort  Port=2  Side=Left
  - : PMIOPort  Port=3  Side=Right
  connections:
  -/RConn1 -- Voltage Sensor/RConn2
  +/RConn1 -- Voltage Sensor/LConn1
  v/RConn1 -- Voltage Sensor/RConn1

== system ODEsim/piLine/M4 ==
  Voltage Sensor : fl_lib/Electrical/Electrical Sensors/Voltage Sensor
  + : PMIOPort  Side=Left
  v : PMIOPort  Port=2  Side=Left
  - : PMIOPort  Port=3  Side=Right
  connections:
  v/RConn1 -- Voltage Sensor/RConn1
  +/RConn1 -- Voltage Sensor/LConn1
  -/RConn1 -- Voltage Sensor/RConn2
